simulink model "hyd_hyb_2_int_cont_Final_AMT"  (R2013b)
settings: Solver=ode4  StartTime=0  StopTime=3005  FixedStep=0.01  MaxStep=.4  RelTol=1e-8
InitFcn:
  | const_3_new
values from neighbouring files (symbols this model uses):
  Af = 6.3    [brk_enrg.m]    (also in brk_enrg_1.m)
  BSFC_906_205 = [3.5684 4.3466 5.1668 6.0769 6.988 7.8992 8.8104 9.7336 10.8548 11.9809 13.1112 14.2571 ... (663 elements, 39x17)]    [BSFC_map_906_205.mat]
  Cd = 0.55    [brk_enrg.m]    (also in brk_enrg_1.m)
  den = 1.202    [brk_enrg.m]    (also in brk_enrg_1.m)
  fr = 0.01    [brk_enrg.m]    (also in brk_enrg_1.m)
undefined symbols (not defined in the file or in its folder): clutchRise, down_spd_2, down_spd_3, down_spd_4, down_spd_c, Driving_Cycle, fuel_density, gearshift, I_wheel, Idle_spd_eng_906, M1_hydr, p_v_15, pmax_125, qv_125, Rw, sec_eng_sfc_map, T0, T1, T_max_906, T_min, TC_spd_ratio_max, teta_new_10, torque_convertor, Twait, up_spd_1, up_spd_2, up_spd_3, up_spd_c, v_p_10, v_p_15, v_p_5
libraries: neural x1742, fl_lib x43, nesl_utility x30, sdl_lib x14, simulink x4, simulink_need_slupdate x1
(part 14 of 26)

== system hyd_hyb_2_int_cont_Final_AMT/controller1/optimized controller/SOC upper 0.5/SOC upper 0.6/SOC under 0.7/net_col_a_b_6_7/Layer 2/LW{2,1} ==
  "ad{2,1}" : Inport  PortDimensions=15
  "IW{2,1}(1,:)'" : Constant  Value=[0.78053014166343337;0.29204864759646343;0.60078593871991481;0.19930621440626281;-0.6417603988784718;0.33501662440183899;-0.039320692942124112;-0.17818770289629898;0.070466356241360939;-0.66502927238801224;-0.32842903100439153;0.20158473933058277;-0.60401576805008483;0.63057683991132762;0.46880386290573689]
  "IW{2,1}(10,:)'" : Constant  Value=[-0.30542783009719876;-0.066026211922728451;-0.35100377549008915;-0.6458951406528961;0.6850695817633381;0.050282872485727714;-0.44195196962407135;-0.71948403799261362;0.4935632179122752;0.200989642702293;-0.64740412469558006;-0.30623454495757785;-0.13820376368835832;0.62066412214227229;0.17661621326669177]
  "IW{2,1}(11,:)'" : Constant  Value=[0.55562311688590493;0.29292130824353235;-0.24419391791645448;0.076845837964054267;0.60243335325886216;0.80506769153284086;-0.62258315480057702;-0.70181319186512137;0.60049372064453754;-0.12668155594586542;0.2553065093083014;-0.018042964286782859;0.4246140714880226;0.28651937946006795;-0.68228531233739165]
  "IW{2,1}(12,:)'" : Constant  Value=[0.44416805338287024;-0.41349849912235709;-0.2531242786660311;0.53251183022901805;-0.32829808880094952;-0.051197223412570408;0.27404319415393802;0.1490633159542053;-0.54269341475467026;0.5760741998500214;-0.0089493484532183008;-0.59671259088667472;-0.47994730366761462;0.71734359409363657;-0.30739574144086385]
  "IW{2,1}(13,:)'" : Constant  Value=[0.15982120682309786;-0.53065964935234877;0.20469363114772193;-0.72220585278335447;0.25545679685766259;0.46446907755731137;-0.73279447878498261;0.33655378845066519;0.61218591810154344;0.32806776740226229;-0.40812289383238065;-0.53302040536360651;0.38560033802278365;-0.11260146758867617;-0.18156471207988037]
  "IW{2,1}(14,:)'" : Constant  Value=[0.45939822916667666;-0.10380478907464295;0.87572221134442962;0.55983631125429267;-0.6443085799942323;-0.438658480407774;0.1355138270898946;0.36487304620458905;0.16874931498791979;-0.61715910709633148;0.036742549389975593;0.57010417817567027;0.25068623188517275;0.21237791145242596;-0.39946964234245058]
  "IW{2,1}(15,:)'" : Constant  Value=[0.47915172534700973;0.27255790315287942;0.22442881940530401;0.7046931447803112;-0.42347258475423294;0.20776969353826535;-0.0029235768347837467;0.54017509885430626;0.3689196436222304;-0.34046687310245394;-0.30779540105947106;0.095620590251799184;-0.71005195669820909;0.14618524222178611;-0.67403650577607799]
  "IW{2,1}(16,:)'" : Constant  Value=[0.17904077524511536;-0.24759703073580216;0.15354503510687395;0.29995487676372212;-0.83029993499257815;-0.54876470636749908;0.1205063780077144;0.21307832098136134;-0.35023088138505193;0.63285269778590514;-0.36348606773018222;0.12068316900064874;-0.58955228467198162;-0.79539775287905845;-0.48918703494261001]
  "IW{2,1}(17,:)'" : Constant  Value=[-0.34794065988557443;0.55219523589663044;0.5143001603488625;-0.22641708498023344;0.50619738437069095;-0.43357233865330164;-0.31471975107068806;0.44989222134038892;0.020171528379251125;-0.49879442794679685;0.69495060944475706;0.18416728478369501;-0.64194628926812813;-0.44892717349124922;-0.02992035603949263]
  "IW{2,1}(18,:)'" : Constant  Value=[0.30331895611664617;-0.12851315036563801;-0.53462584873971397;-0.46371560949317192;0.13988007049048459;-0.40859791032484338;-0.79681484818945858;-0.016377073182308237;-0.38358662973594859;0.35861055563777722;-0.6496507650902974;-0.62090439723521351;0.076840851410475489;0.63048254223125022;-0.17904919957529017]
  "IW{2,1}(19,:)'" : Constant  Value=[0.42136534934876768;-0.094259274675504004;0.38571921238709894;-0.25975786849453808;0.27980642914644399;0.25103986804488559;-0.60536259986501006;-0.77907072761843155;0.36344966644543175;0.37496372736772582;0.21893946612478141;-0.36281736420872207;-0.12483282318384557;0.44599078258141628;0.85808382076373013]
  "IW{2,1}(2,:)'" : Constant  Value=[0.17575627492329865;0.64661608900825296;0.42137302105518887;-0.44175042575697759;-0.4997020622910609;-0.24150363000577296;-0.54227929869906655;-0.030900429610183539;-0.89489142801219335;-0.63703091125729705;0.42177423558752708;0.27215046474187243;-0.34698223791053751;0.66722016984498034;-0.0061883428480007099]
  "IW{2,1}(20,:)'" : Constant  Value=[0.63439636960799195;-0.0079849099056435568;-0.29312179824428075;-0.11661323059913765;-0.059062754602998473;0.42181160788884509;-0.354936423434419;-0.79002736369917981;0.68314796367141561;-0.31626111931508516;0.18488824411974616;-0.62932262549817952;-0.0026698991954153626;0.65819654748933976;0.29779376842812089]
  "IW{2,1}(3,:)'" : Constant  Value=[-0.12217583136931578;-0.63766103817813291;0.43517835173933522;0.63293446833365052;-0.52860303763913297;-0.76213283901609874;0.14191460170451217;-0.11103439622102566;0.73461022496268757;-0.0047405745337899272;-0.009656240798445315;0.37011754169114702;0.47350620034919455;-0.46645161835048304;0.43334555205260494]
  "IW{2,1}(4,:)'" : Constant  Value=[-0.2005453869405778;0.64893992256903765;0.70402350909180733;0.35856884485351742;0.18900524632612653;0.28089732179910709;0.021155364578440541;0.01900818391730108;0.61684363687319277;-0.22545734121955546;-0.77847633978361408;0.5923575841709301;-0.35224507873924205;0.42076565418116368;0.18895037854545177]
  "IW{2,1}(5,:)'" : Constant  Value=[-0.5873832365212881;0.5870340061374888;0.51879881610097367;0.20306262712379949;0.58198472367706588;-0.088541754224339103;0.60265415473813688;-0.49303371593315082;-0.49232604461319407;-0.15524092257009237;-0.059729873946896203;-0.59340865182430658;0.38715282547449376;0.12736848545340604;-0.43961102624085946]
  "IW{2,1}(6,:)'" : Constant  Value=[0.13736446076866377;0.47148069258784503;-0.35630029659432555;-0.48574242196604062;0.69829640255595016;0.74119954705384339;0.70446786249556448;-0.54164780220432129;0.027062046923033337;-0.32813978317482456;0.20312485406186492;0.20471190638401837;-0.27774373666160662;-0.29877561054994162;0.68667414286446171]
  "IW{2,1}(7,:)'" : Constant  Value=[-0.57571717755453788;-0.0059675488607752293;0.66823977219967612;-0.13032210666990385;-0.39771462827240905;0.70065202775840507;0.24651655595225383;0.15421059694834863;-0.45372541376902564;0.45027176851886697;0.26911175175141044;0.66136745379510065;0.46051315523515801;0.44007352575074449;0.3291262643302636]
  "IW{2,1}(8,:)'" : Constant  Value=[-0.13468571110448263;-0.72001015586532779;0.83168168898079686;0.051300439567951731;-0.29413778931308698;0.35588121434291087;0.13832855947874259;-0.52825182599939458;-0.22776972548979266;0.095012379619955262;-0.64412283600444264;0.033898997348194994;0.65343908042137089;0.36369099742500133;-0.11910178969771282]
  "IW{2,1}(9,:)'" : Constant  Value=[0.26997185648634625;0.26405799369778199;-0.37801464377310512;0.68067072958776387;0.63431596479861185;0.21053904943579516;0.50234312720935115;-0.55377188611462114;-0.46914553861348829;-0.55620160039681665;0.020771550954338174;0.29202998467294183;-0.31675450684928891;0.58500586597730353;0.44301086121313571]
  Mux : Mux  Inputs=20
  dotprod{1..20} (20 alike) : neural/Weight Functions/dotprod
  "lz{2,1}" : Outport
  wires:
  Mux/1 -> "lz{2,1}"/1
  dotprod20/1 -> Mux/20
  "IW{2,1}(20,:)'"/1 -> dotprod20/1
  dotprod19/1 -> Mux/19
  "IW{2,1}(19,:)'"/1 -> dotprod19/1
  dotprod18/1 -> Mux/18
  "IW{2,1}(18,:)'"/1 -> dotprod18/1
  dotprod17/1 -> Mux/17
  "IW{2,1}(17,:)'"/1 -> dotprod17/1
  dotprod16/1 -> Mux/16
  "IW{2,1}(16,:)'"/1 -> dotprod16/1
  dotprod15/1 -> Mux/15
  "IW{2,1}(15,:)'"/1 -> dotprod15/1
  dotprod14/1 -> Mux/14
  "IW{2,1}(14,:)'"/1 -> dotprod14/1
  dotprod13/1 -> Mux/13
  "IW{2,1}(13,:)'"/1 -> dotprod13/1
  dotprod12/1 -> Mux/12
  "IW{2,1}(12,:)'"/1 -> dotprod12/1
  dotprod11/1 -> Mux/11
  "IW{2,1}(11,:)'"/1 -> dotprod11/1
  dotprod10/1 -> Mux/10
  "IW{2,1}(10,:)'"/1 -> dotprod10/1
  dotprod9/1 -> Mux/9
  "IW{2,1}(9,:)'"/1 -> dotprod9/1
  dotprod8/1 -> Mux/8
  "IW{2,1}(8,:)'"/1 -> dotprod8/1
  dotprod7/1 -> Mux/7
  "IW{2,1}(7,:)'"/1 -> dotprod7/1
  dotprod6/1 -> Mux/6
  "IW{2,1}(6,:)'"/1 -> dotprod6/1
  dotprod5/1 -> Mux/5
  "IW{2,1}(5,:)'"/1 -> dotprod5/1
  dotprod4/1 -> Mux/4
  "IW{2,1}(4,:)'"/1 -> dotprod4/1
  dotprod3/1 -> Mux/3
  "IW{2,1}(3,:)'"/1 -> dotprod3/1
  dotprod2/1 -> Mux/2
  "IW{2,1}(2,:)'"/1 -> dotprod2/1
  dotprod1/1 -> Mux/1
  "ad{2,1}"/1 -> dotprod20/2, dotprod19/2, dotprod18/2, dotprod17/2, dotprod16/2, dotprod15/2, dotprod14/2, dotprod13/2, dotprod12/2, dotprod11/2, dotprod10/2, dotprod9/2, dotprod8/2, dotprod7/2, dotprod6/2, dotprod5/2, dotprod4/2, dotprod3/2, dotprod2/2, dotprod1/2
  "IW{2,1}(1,:)'"/1 -> dotprod1/1

== system hyd_hyb_2_int_cont_Final_AMT/controller1/optimized controller/SOC upper 0.5/SOC upper 0.6/SOC under 0.7/net_col_a_b_6_7/Layer 3/Delays 1 ==
  "p{3}" : Inport  PortDimensions=20
  mux : Mux  Inputs=1
  "pd{3,2}" : Outport
  wires:
  mux/1 -> "pd{3,2}"/1
  "p{3}"/1 -> mux/1

== system hyd_hyb_2_int_cont_Final_AMT/controller1/optimized controller/SOC upper 0.5/SOC upper 0.6/SOC under 0.7/net_col_a_b_6_7/Layer 3/LW{3,2} ==
  "ad{3,2}" : Inport  PortDimensions=20
  "IW{3,2}(1,:)'" : Constant  Value=[-0.34903886609399382;1.06705366788284;-0.63069522814965984;0.43720033513892198;-0.11763112400213262;-0.71855053606900632;-0.34692052449521499;-0.46231517262753691;1.0151944900739838;-0.45066968253451173;1.1029155009020308;-0.37855254899971402;0.025219381776951783;-0.56955532675060594;0.74416374807652608;0.63806693225984767;-0.10748465748831162;-0.72740367544789852;0.024756316136680077;0.39060697940746125]
  Mux : Mux  Inputs=1
  dotprod1 : neural/Weight Functions/dotprod
  "lz{3,2}" : Outport
  wires:
  Mux/1 -> "lz{3,2}"/1
  dotprod1/1 -> Mux/1
  "ad{3,2}"/1 -> dotprod1/2
  "IW{3,2}(1,:)'"/1 -> dotprod1/1

== system hyd_hyb_2_int_cont_Final_AMT/controller1/optimized controller/SOC upper 0.5/SOC upper 0.6/SOC under 0.7/net_col_e_f_6_7/Layer 1/Delays 1 ==
  "p{1}" : Inport  PortDimensions=2
  mux : Mux  Inputs=1
  "pd{1,1}" : Outport
  wires:
  mux/1 -> "pd{1,1}"/1
  "p{1}"/1 -> mux/1

== system hyd_hyb_2_int_cont_Final_AMT/controller1/optimized controller/SOC upper 0.5/SOC upper 0.6/SOC under 0.7/net_col_e_f_6_7/Layer 1/IW{1,1} ==
  "pd{1,1}" : Inport  PortDimensions=2
  "IW{1,1}(1,:)'" : Constant  Value=[4.6180581373625786;-7.5513248281960692]
  "IW{1,1}(10,:)'" : Constant  Value=[-7.3411562704687192;-4.9409171823199811]
  "IW{1,1}(11,:)'" : Constant  Value=[1.2697021096317962;-8.7667698979188291]
  "IW{1,1}(12,:)'" : Constant  Value=[8.2105168529205113;-3.2999808705776745]
  "IW{1,1}(13,:)'" : Constant  Value=[8.00239705929339;-3.7896987598116452]
  "IW{1,1}(14,:)'" : Constant  Value=[-3.1920512868443462;8.2769860449078756]
  "IW{1,1}(15,:)'" : Constant  Value=[-8.6415814148069394;-1.9030849843180959]
  "IW{1,1}(16,:)'" : Constant  Value=[-0.3539411796819058;-8.8441255202432831]
  "IW{1,1}(17,:)'" : Constant  Value=[-7.3859013101945274;4.8793595183912082]
  "IW{1,1}(18,:)'" : Constant  Value=[7.7137987954855012;4.3463573532002338]
  "IW{1,1}(19,:)'" : Constant  Value=[-3.3006613050491569;8.2142066761667056]
  "IW{1,1}(2,:)'" : Constant  Value=[-8.0361960972906665;-3.724407320242006]
  "IW{1,1}(20,:)'" : Constant  Value=[-6.8829766745436949;-5.5692487475075403]
  "IW{1,1}(21,:)'" : Constant  Value=[2.4714071551610424;-8.5004348942069683]
  "IW{1,1}(22,:)'" : Constant  Value=[7.6310179912154803;4.4909506530540781]
  "IW{1,1}(23,:)'" : Constant  Value=[5.9240299449083782;6.5806465278605542]
  "IW{1,1}(24,:)'" : Constant  Value=[6.9897101383703131;-5.5420246789012229]
  "IW{1,1}(25,:)'" : Constant  Value=[-1.0535387549303452;-8.7946441386292999]
  "IW{1,1}(26,:)'" : Constant  Value=[-8.2305860437938865;3.0834290009841205]
  "IW{1,1}(27,:)'" : Constant  Value=[2.9220969367198872;8.359129848716611]
  "IW{1,1}(28,:)'" : Constant  Value=[0.78649843915295814;-8.8067333816792974]
  "IW{1,1}(29,:)'" : Constant  Value=[6.862179573851594;5.5951061158057769]
  "IW{1,1}(3,:)'" : Constant  Value=[7.2513831806494382;-5.0791324458970761]
  "IW{1,1}(30,:)'" : Constant  Value=[3.6501584030846903;8.0652553752255134]
  "IW{1,1}(31,:)'" : Constant  Value=[-2.5524936658049273;8.4641721866602815]
  "IW{1,1}(32,:)'" : Constant  Value=[2.5001075311498955;-8.5082754822093225]
  "IW{1,1}(33,:)'" : Constant  Value=[-7.8765128218500298;-4.0217909102733653]
  "IW{1,1}(34,:)'" : Constant  Value=[-7.9423905495076577;3.9175438683997994]
  "IW{1,1}(35,:)'" : Constant  Value=[7.0501043369622485;5.3308743978689366]
  "IW{1,1}(36,:)'" : Constant  Value=[3.7966677997716936;7.9942931542438576]
  "IW{1,1}(37,:)'" : Constant  Value=[-7.5643449957345235;4.6037891808307823]
  "IW{1,1}(38,:)'" : Constant  Value=[0.9358380449019762;8.7912415356316984]
  "IW{1,1}(39,:)'" : Constant  Value=[-2.2880473566171591;8.5583565392320597]
  "IW{1,1}(4,:)'" : Constant  Value=[-8.606945132383883;2.0740017422588424]
  "IW{1,1}(40,:)'" : Constant  Value=[-3.9073322523914027;7.9452744576412009]
  "IW{1,1}(5,:)'" : Constant  Value=[0.63432776663309298;-8.8021870561531497]
  "IW{1,1}(6,:)'" : Constant  Value=[-0.2733127448645003;-8.8604684481923091]
  "IW{1,1}(7,:)'" : Constant  Value=[-0.89606946382595276;8.8022472216947918]
  "IW{1,1}(8,:)'" : Constant  Value=[3.4953292810936971;-8.1719817954370892]
  "IW{1,1}(9,:)'" : Constant  Value=[-0.33420269573780609;8.8625107908198935]
  Mux : Mux  Inputs=40
  dotprod{1..40} (40 alike) : neural/Weight Functions/dotprod
  "iz{1,1}" : Outport
  wires:
  Mux/1 -> "iz{1,1}"/1
  dotprod40/1 -> Mux/40
  "IW{1,1}(40,:)'"/1 -> dotprod40/1
  dotprod39/1 -> Mux/39
  "IW{1,1}(39,:)'"/1 -> dotprod39/1
  dotprod38/1 -> Mux/38
  "IW{1,1}(38,:)'"/1 -> dotprod38/1
  dotprod37/1 -> Mux/37
  "IW{1,1}(37,:)'"/1 -> dotprod37/1
  dotprod36/1 -> Mux/36
  "IW{1,1}(36,:)'"/1 -> dotprod36/1
  dotprod35/1 -> Mux/35
  "IW{1,1}(35,:)'"/1 -> dotprod35/1
  dotprod34/1 -> Mux/34
  "IW{1,1}(34,:)'"/1 -> dotprod34/1
  dotprod33/1 -> Mux/33
  "IW{1,1}(33,:)'"/1 -> dotprod33/1
  dotprod32/1 -> Mux/32
  "IW{1,1}(32,:)'"/1 -> dotprod32/1
  dotprod31/1 -> Mux/31
  "IW{1,1}(31,:)'"/1 -> dotprod31/1
  dotprod30/1 -> Mux/30
  "IW{1,1}(30,:)'"/1 -> dotprod30/1
  dotprod29/1 -> Mux/29
  "IW{1,1}(29,:)'"/1 -> dotprod29/1
  dotprod28/1 -> Mux/28
  "IW{1,1}(28,:)'"/1 -> dotprod28/1
  dotprod27/1 -> Mux/27
  "IW{1,1}(27,:)'"/1 -> dotprod27/1
  dotprod26/1 -> Mux/26
  "IW{1,1}(26,:)'"/1 -> dotprod26/1
  dotprod25/1 -> Mux/25
  "IW{1,1}(25,:)'"/1 -> dotprod25/1
  dotprod24/1 -> Mux/24
  "IW{1,1}(24,:)'"/1 -> dotprod24/1
  dotprod23/1 -> Mux/23
  "IW{1,1}(23,:)'"/1 -> dotprod23/1
  dotprod22/1 -> Mux/22
  "IW{1,1}(22,:)'"/1 -> dotprod22/1
  dotprod21/1 -> Mux/21
  "IW{1,1}(21,:)'"/1 -> dotprod21/1
  dotprod20/1 -> Mux/20
  "IW{1,1}(20,:)'"/1 -> dotprod20/1
  dotprod19/1 -> Mux/19
  "IW{1,1}(19,:)'"/1 -> dotprod19/1
  dotprod18/1 -> Mux/18
  "IW{1,1}(18,:)'"/1 -> dotprod18/1
  dotprod17/1 -> Mux/17
  "IW{1,1}(17,:)'"/1 -> dotprod17/1
  dotprod16/1 -> Mux/16
  "IW{1,1}(16,:)'"/1 -> dotprod16/1
  dotprod15/1 -> Mux/15
  "IW{1,1}(15,:)'"/1 -> dotprod15/1
  dotprod14/1 -> Mux/14
  "IW{1,1}(14,:)'"/1 -> dotprod14/1
  dotprod13/1 -> Mux/13
  "IW{1,1}(13,:)'"/1 -> dotprod13/1
  dotprod12/1 -> Mux/12
  "IW{1,1}(12,:)'"/1 -> dotprod12/1
  dotprod11/1 -> Mux/11
  "IW{1,1}(11,:)'"/1 -> dotprod11/1
  dotprod10/1 -> Mux/10
  "IW{1,1}(10,:)'"/1 -> dotprod10/1
  dotprod9/1 -> Mux/9
  "IW{1,1}(9,:)'"/1 -> dotprod9/1
  dotprod8/1 -> Mux/8
  "IW{1,1}(8,:)'"/1 -> dotprod8/1
  dotprod7/1 -> Mux/7
  "IW{1,1}(7,:)'"/1 -> dotprod7/1
  dotprod6/1 -> Mux/6
  "IW{1,1}(6,:)'"/1 -> dotprod6/1
  dotprod5/1 -> Mux/5
  "IW{1,1}(5,:)'"/1 -> dotprod5/1
  dotprod4/1 -> Mux/4
  "IW{1,1}(4,:)'"/1 -> dotprod4/1
  dotprod3/1 -> Mux/3
  "IW{1,1}(3,:)'"/1 -> dotprod3/1
  dotprod2/1 -> Mux/2
  "IW{1,1}(2,:)'"/1 -> dotprod2/1
  dotprod1/1 -> Mux/1
  "pd{1,1}"/1 -> dotprod40/2, dotprod39/2, dotprod38/2, dotprod37/2, dotprod36/2, dotprod35/2, dotprod34/2, dotprod33/2, dotprod32/2, dotprod31/2, dotprod30/2, dotprod29/2, dotprod28/2, dotprod27/2, dotprod26/2, dotprod25/2, dotprod24/2, dotprod23/2, dotprod22/2, dotprod21/2, dotprod20/2, dotprod19/2, dotprod18/2, dotprod17/2, dotprod16/2, dotprod15/2, dotprod14/2, dotprod13/2, dotprod12/2, dotprod11/2, dotprod10/2, dotprod9/2, dotprod8/2, dotprod7/2, dotprod6/2, dotprod5/2, dotprod4/2, dotprod3/2, dotprod2/2, dotprod1/2
  "IW{1,1}(1,:)'"/1 -> dotprod1/1

== system hyd_hyb_2_int_cont_Final_AMT/controller1/optimized controller/SOC upper 0.5/SOC upper 0.6/SOC under 0.7/net_col_e_f_6_7/Layer 2/Delays 1 ==
  "p{2}" : Inport  PortDimensions=40
  mux : Mux  Inputs=1
  "pd{2,1}" : Outport
  wires:
  mux/1 -> "pd{2,1}"/1
  "p{2}"/1 -> mux/1
